simulink library "V8SC_controls"  (R2026a)
settings: Solver=VariableStepAuto
libraries: $bdroot x4, matrix_library x2
settings Model: Creator=lholliday  LastModifiedBy=lholliday

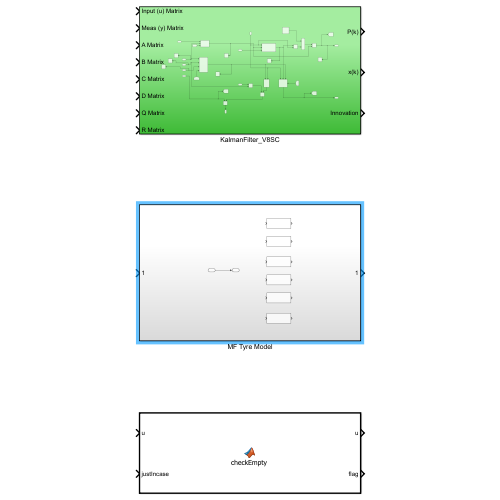
[thumbnail: Simulink's stored preview of the top-level diagram]
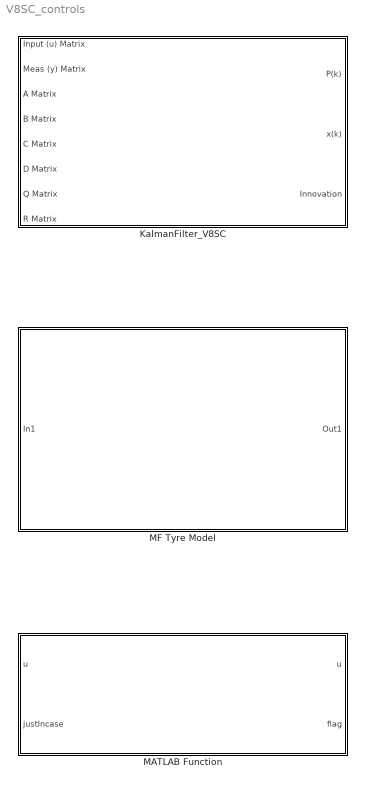
== system V8SC_controls ==
  KalmanFilter_V8SC : Subsystem
  MATLAB Function : MATLAB Function  TreatAsAtomicUnit=on
  MF Tyre Model : Subsystem

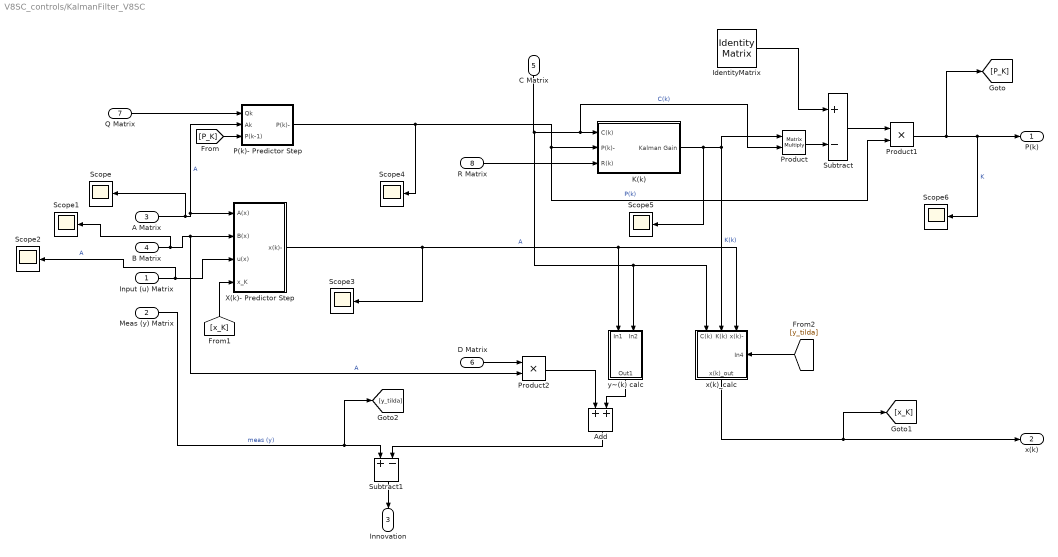
== system V8SC_controls/KalmanFilter_V8SC ==
  Input (u) Matrix : Inport
  Meas (y) Matrix : Inport  Port=2
  A Matrix : Inport  Port=3
  B Matrix : Inport  Port=4
  C Matrix : Inport  Port=5
  D Matrix : Inport  Port=6
  Q Matrix : Inport  Port=7
  R Matrix : Inport  Port=8
  Add : Sum
  IdentityMatrix : IdentityMatrix  OutputDimensions=2
  K(k) : Subsystem
  P(k)- Predictor Step : Subsystem
  Product : Product  Multiplication=Matrix(*)
  Product1 : Product
  Product2 : Product
  Scope{,1..6} (7 alike) : Scope
      Scope settings: ActiveDisplayYMinimum=-2708.7005445946597  ActiveDisplayYMaximum=17569.63847850831  DataLoggingVariableName=ScopeData16
      Scope1 settings: ActiveDisplayYMinimum=-76.902863771048189  ActiveDisplayYMaximum=81.800535438034714  DataLoggingVariableName=ScopeData17
      Scope2 settings: ActiveDisplayYMinimum=-0.35626533356334256  ActiveDisplayYMaximum=0.37895461383926876  DataLoggingVariableName=ScopeData18
      Scope3 settings: ActiveDisplayYMinimum=-1  ActiveDisplayYMaximum=1  DataLoggingVariableName=ScopeData19
      Scope4 settings: ActiveDisplayYMinimum=-2708.7005445946597  ActiveDisplayYMaximum=17569.63847850831  DataLoggingVariableName=ScopeData16
      Scope5 settings: ActiveDisplayYMinimum=-2708.7005445946597  ActiveDisplayYMaximum=17569.63847850831  DataLoggingVariableName=ScopeData17
      Scope6 settings: ActiveDisplayYMinimum=-2708.7005445946597  ActiveDisplayYMaximum=17569.63847850831  DataLoggingVariableName=ScopeData18
  Subtract : Sum  Inputs=+-
  Subtract1 : Sum  Inputs=+-
  X(k)- Predictor Step : Subsystem
  x(k)_calc : Subsystem
      settings: PortSchema="{\"entries\":[{\"content\":{\"sides\":[{\"content\":{\"connectorIds\":[\"In1\",\"In2\",\"In3\"]},\"type\":\"ConnectorPlacement.EquallySpacedRectSide\",\"uuid\":\"9798f8d0-e1e5-4082-961b-6e38066891ac\"},{\"content\":{\"connectorIds\":[\"Out1\"],\"side\":\"RIGHT\"},\"type\":\"ConnectorPlacement.EquallySpacedRectSide\",\"uuid\":\"85739a9d-0a70-4322-86b9-e4ddcc6280df\"},{\"content\":{\"side\":\"TOP\"},\"type\":\"ConnectorPlacement.EquallySpacedRectSide\",\"uuid\":\"b405db1d-aea8-46b4-b741-29e757833e0c\"},{\"content\":{\"connectorIds\":[\"In4\"],\"side\":\"BOTTOM\"},\"type\":\"ConnectorPlacement.EquallySpacedRectSide\",\"uuid\":\"98479f7e-2eaa-4af4-b745-0172a8769d4f\"}]},\"type\":\"ConnectorPlacement.EquallySpacedConnector\",\"uuid\":\"fea33aa2-baa4-4ea5-bbbc-a180d2a37d17\"}],\"packageUris\":[\"http://schema.mathworks.com/mf0/Connector/R2020b\"],\"version\":\"1.0\"}"
  y~(k) calc : Subsystem
  P(k) : Outport
  x(k) : Outport  Port=2
  Innovation : Outport  Port=3
  wires:
  Add/1 -> Subtract1/2
  Product2/1 -> Add/1
  D Matrix/1 -> Product2/1
  X(k)- Predictor Step/1(x(k)-) -> x(k)_calc/3(x(k)-), y~(k) calc/1(In1), Scope3/1  "A"
  Input (u) Matrix/1 -> X(k)- Predictor Step/3(u(x)), Scope2/1  "A"
  B Matrix/1 -> X(k)- Predictor Step/2(B(x)), Product2/2, Scope1/1  "A"
  A Matrix/1 -> X(k)- Predictor Step/1(A(x)), P(k)- Predictor Step/2(Ak), Scope/1  "A"
  C Matrix/1 -> y~(k) calc/2(In2), x(k)_calc/1(C(k)), K(k)/1(C(k)), Product/2  "C(k)"
  P(k)- Predictor Step/1(P(k)-) -> Product1/2, K(k)/2(P(k)-), Scope4/1  "P(k)"
  Q Matrix/1 -> P(k)- Predictor Step/1(Qk)
  K(k)/1(Kalman Gain) -> x(k)_calc/2(K(k)), Product/1, Scope5/1  "K(k)"
  Product/1 -> Subtract/2
  IdentityMatrix/1 -> Subtract/1
  Subtract/1 -> Product1/1
  Product1/1 -> [P_K], P(k)/1, Scope6/1  "K"
  x(k)_calc/1(x(k)_out) -> [x_K], x(k)/1
  y~(k) calc/1(Out1) -> Add/2
  Meas (y) Matrix/1 -> [y_tilda], Subtract1/1  "meas (y)"
  [P_K] -> P(k)- Predictor Step/3(P(k-1))
  [x_K] -> X(k)- Predictor Step/4(x_K)
  R Matrix/1 -> K(k)/3(R(k))
  [y_tilda] -> x(k)_calc/4(In4)
  Subtract1/1 -> Innovation/1

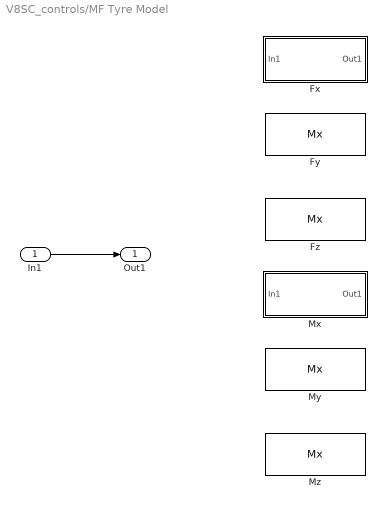
== system V8SC_controls/MF Tyre Model ==
  In1 : Inport
  Fx : Subsystem  AncestorBlock=V8SC_controls/MF Tyre Model/Mx
  Fy : $bdroot/MF Tyre Model/Mx  SystemSampleTime=-1  VariantActivationTime=update diagram  EmptyChoice=off  PassThrough=off  PassThroughVariantControl=(default)  EmptyChoiceVariantControl=(default)  AllowFlexibleInterface=on  Latency=0  AutoFrameSizeCalculation=off
  Fz : $bdroot/MF Tyre Model/Mx  SystemSampleTime=-1  VariantActivationTime=update diagram  EmptyChoice=off  PassThrough=off  PassThroughVariantControl=(default)  EmptyChoiceVariantControl=(default)  AllowFlexibleInterface=on  Latency=0  AutoFrameSizeCalculation=off
  Mx : Subsystem
  My : $bdroot/MF Tyre Model/Mx  SystemSampleTime=-1  VariantActivationTime=update diagram  EmptyChoice=off  PassThrough=off  PassThroughVariantControl=(default)  EmptyChoiceVariantControl=(default)  AllowFlexibleInterface=on  Latency=0  AutoFrameSizeCalculation=off
  Mz : $bdroot/MF Tyre Model/Mx  SystemSampleTime=-1  VariantActivationTime=update diagram  EmptyChoice=off  PassThrough=off  PassThroughVariantControl=(default)  EmptyChoiceVariantControl=(default)  AllowFlexibleInterface=on  Latency=0  AutoFrameSizeCalculation=off
  Out1 : Outport
  wires:
  In1/1 -> Out1/1

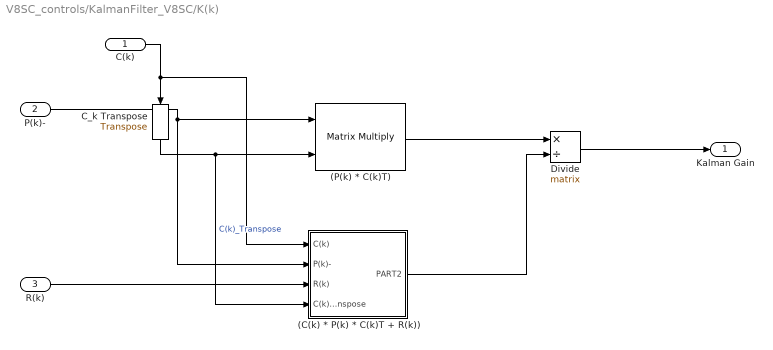
== system V8SC_controls/KalmanFilter_V8SC/K(k) ==
  C(k) : Inport
  P(k)- : Inport  Port=2
  R(k) : Inport  Port=3
  (C(k) * P(k) * C(k)T + R(k)) : Subsystem
  (P(k) * C(k)T) : Product  Multiplication=Matrix(*)
  C_k Transpose : matrix_library/Transpose
  Divide : Product  Inputs=*/  Multiplication=Matrix(*)
  Kalman Gain : Outport
  wires:
  P(k)-/1 -> (P(k) * C(k)T)/1, (C(k) * P(k) * C(k)T + R(k))/2(P(k)-)
  C_k Transpose/1 -> (P(k) * C(k)T)/2, (C(k) * P(k) * C(k)T + R(k))/4(C(k)_Transpose)  "C(k)_Transpose"
  C(k)/1 -> C_k Transpose/1, (C(k) * P(k) * C(k)T + R(k))/1(C(k))
  (C(k) * P(k) * C(k)T + R(k))/1(PART2) -> Divide/2
  R(k)/1 -> (C(k) * P(k) * C(k)T + R(k))/3(R(k))
  (P(k) * C(k)T)/1 -> Divide/1
  Divide/1 -> Kalman Gain/1

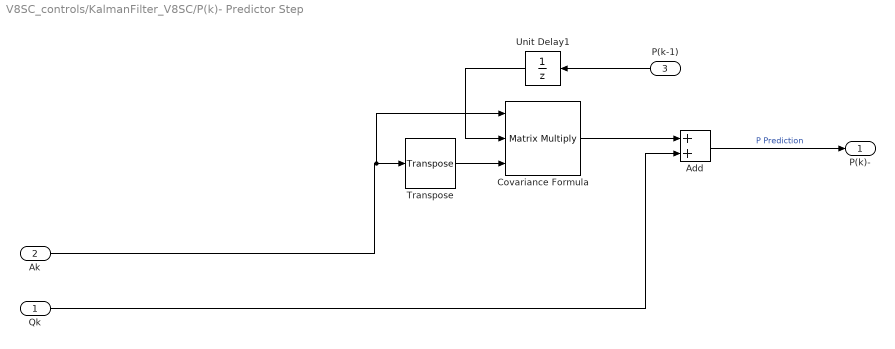
== system V8SC_controls/KalmanFilter_V8SC/P(k)- Predictor Step ==
  Qk : Inport
  Ak : Inport  Port=2
  P(k-1) : Inport  Port=3
  Add : Sum
  Covariance Formula : Product  Inputs=3  Multiplication=Matrix(*)
  Transpose : matrix_library/Transpose
  Unit Delay1 : UnitDelay  SampleTime=-1
  P(k)- : Outport
  wires:
  Unit Delay1/1 -> Covariance Formula/2
  Transpose/1 -> Covariance Formula/3
  Add/1 -> P(k)-/1  "P Prediction"
  Ak/1 -> Covariance Formula/1, Transpose/1
  Qk/1 -> Add/2
  Covariance Formula/1 -> Add/1
  P(k-1)/1 -> Unit Delay1/1

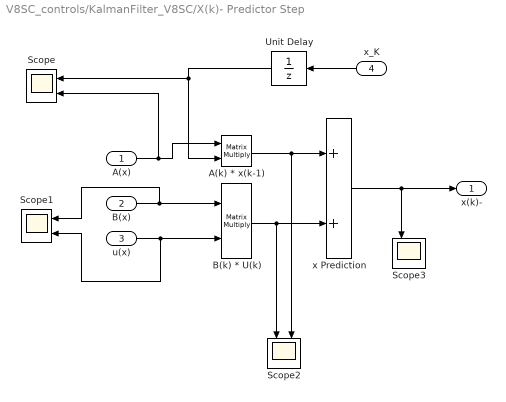
== system V8SC_controls/KalmanFilter_V8SC/X(k)- Predictor Step ==
  A(x) : Inport
  B(x) : Inport  Port=2
  u(x) : Inport  Port=3
  x_K : Inport  Port=4
  A(k) * x(k-1) : Product  Multiplication=Matrix(*)
  B(k) * U(k) : Product  Multiplication=Matrix(*)
  Scope{,1..3} (4 alike) : Scope  NumInputPorts=2
      Scope settings: ActiveDisplayYMinimum=-1  ActiveDisplayYMaximum=1  DataLoggingVariableName=ScopeData20
      Scope1 settings: ActiveDisplayYMinimum=-0.6278212197486237  ActiveDisplayYMaximum=0.7793239513320418  DataLoggingVariableName=ScopeData21
      Scope2 settings: ActiveDisplayYMinimum=-0.939113541591599  ActiveDisplayYMaximum=13.261786146326211  DataLoggingVariableName=ScopeData22
      Scope3 settings: ActiveDisplayYMinimum=-1  ActiveDisplayYMaximum=1  DataLoggingVariableName=ScopeData23
  Unit Delay : UnitDelay  SampleTime=-1
  x Prediction : Sum
  x(k)- : Outport
  wires:
  B(k) * U(k)/1 -> x Prediction/2, Scope2/1
  A(k) * x(k-1)/1 -> x Prediction/1, Scope2/2
  u(x)/1 -> B(k) * U(k)/2, Scope1/2
  B(x)/1 -> B(k) * U(k)/1, Scope1/1
  x Prediction/1 -> x(k)-/1, Scope3/1
  Unit Delay/1 -> Scope/1, A(k) * x(k-1)/2
  A(x)/1 -> A(k) * x(k-1)/1, Scope/2
  x_K/1 -> Unit Delay/1

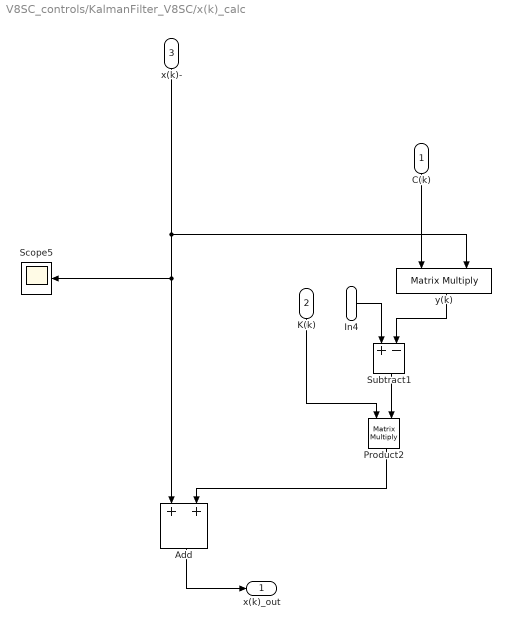
== system V8SC_controls/KalmanFilter_V8SC/x(k)_calc ==
  C(k) : Inport
  K(k) : Inport  Port=2
  x(k)- : Inport  Port=3
  In4 : Inport  Port=4
  Add : Sum
  Product2 : Product  Multiplication=Matrix(*)
  Scope5 : Scope
      settings: ActiveDisplayYMinimum=-2708.7005445946597  ActiveDisplayYMaximum=17569.63847850831  DataLoggingVariableName=ScopeData19
  Subtract1 : Sum  Inputs=+-
  y(k) : Product  Multiplication=Matrix(*)
  x(k)_out : Outport
  wires:
  K(k)/1 -> Product2/1
  y(k)/1 -> Subtract1/2
  x(k)-/1 -> y(k)/2, Add/1, Scope5/1
  Product2/1 -> Add/2
  C(k)/1 -> y(k)/1
  In4/1 -> Subtract1/1
  Subtract1/1 -> Product2/2
  Add/1 -> x(k)_out/1

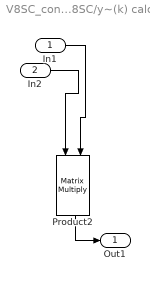
== system V8SC_controls/KalmanFilter_V8SC/y~(k) calc ==
  In1 : Inport
  In2 : Inport  Port=2
  Product2 : Product  Multiplication=Matrix(*)
  Out1 : Outport
  wires:
  In1/1 -> Product2/2
  Product2/1 -> Out1/1
  In2/1 -> Product2/1

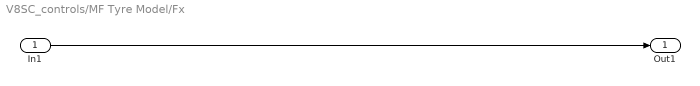
== system V8SC_controls/MF Tyre Model/Fx ==
  In1 : Inport
  Out1 : Outport
  wires:
  In1/1 -> Out1/1

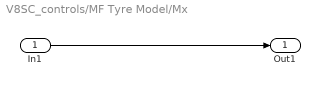
== system V8SC_controls/MF Tyre Model/Mx ==
  In1 : Inport
  Out1 : Outport
  wires:
  In1/1 -> Out1/1

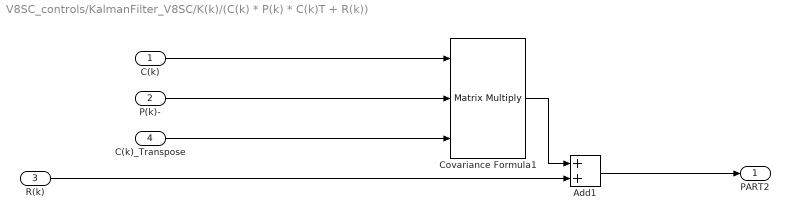
== system V8SC_controls/KalmanFilter_V8SC/K(k)/(C(k) * P(k) * C(k)T + R(k)) ==
  C(k) : Inport
  P(k)- : Inport  Port=2
  R(k) : Inport  Port=3
  C(k)_Transpose : Inport  Port=4
  Add1 : Sum
  Covariance Formula1 : Product  Inputs=3  Multiplication=Matrix(*)
  PART2 : Outport
  wires:
  P(k)-/1 -> Covariance Formula1/2
  Covariance Formula1/1 -> Add1/1
  C(k)/1 -> Covariance Formula1/1
  R(k)/1 -> Add1/2
  C(k)_Transpose/1 -> Covariance Formula1/3
  Add1/1 -> PART2/1

== matlab function V8SC_controls/MATLAB Function ==
  data: u input; u output; justIncase input; flag output
function [u, flag] = checkEmpty(u, justIncase)
    if isempty(u)
        u = u; % Variable is empty
        flag = 0; 
    else
        u = justIncase; % Variable contains data
        flag = 1;
    end
end
